simulink model "untitled2"  (R2018b)
settings: Solver=VariableStepAuto  StartTime=0.0  StopTime=3  RelTol=1e-3
libraries: commfilt2 x2, commsink2 x1, commrandsrc3 x1
settings Model: Creator=nhat  LastModifiedBy=nhat

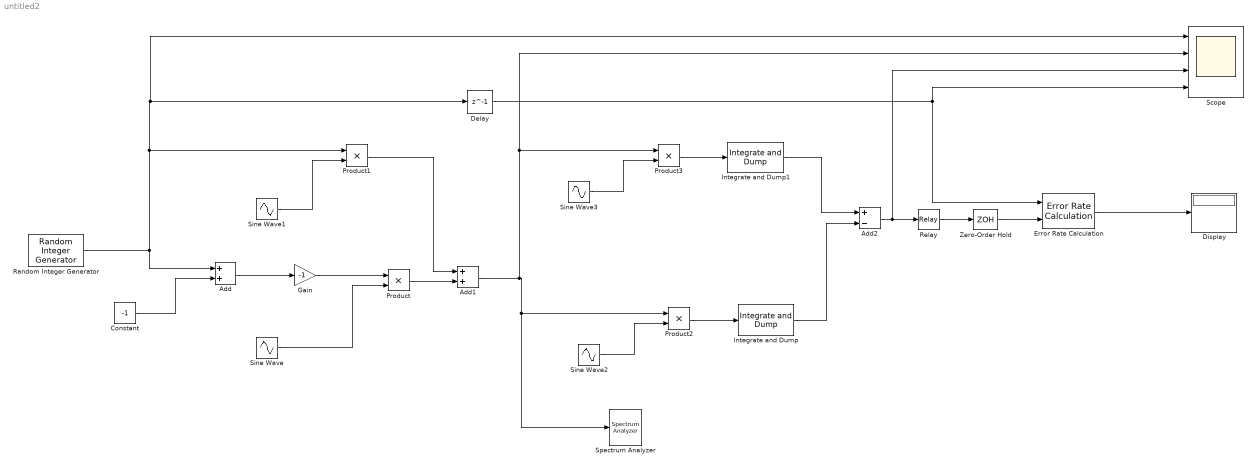
== system untitled2 ==
  Add : Sum
  Add1 : Sum
  Add2 : Sum  Inputs=+-
  Constant : Constant  Value=-1
  Delay : Delay  DelayLength=1
  Display : Display
  Error Rate Calculation : commsink2/Error Rate Calculation  N=0  st_delay=0  cp_mode=Entire frame  subframe=[]  PMode=Port  WsName=ErrorVec  RsMode2=off  stop=off  numErr=100  maxBits=1e6
  Gain : Gain  Gain=-1
  Integrate and Dump : commfilt2/Integrate and Dump  obssamples=100  offsetsamples=0  nodump=off  roundingMode=Floor  overflowMode=off  outputDataTypeStr=Inherit: Same as accumulator  outputLastDataTypeStr=Inherit: Same as accumulator
      settings: SourceProductName=Communications System Toolbox
  Integrate and Dump1 : commfilt2/Integrate and Dump  obssamples=100  offsetsamples=0  nodump=off  roundingMode=Floor  overflowMode=off  outputDataTypeStr=Inherit: Same as accumulator  outputLastDataTypeStr=Inherit: Same as accumulator
      settings: SourceProductName=Communications System Toolbox
  Product{,1..3} (4 alike) : Product
  Random Integer Generator : commrandsrc3/Random Integer Generator  SetSize=2  SeedSource=Auto  Seed=0  SampleTime=1/1000  SamplesPerFrame=1  OutputDataType=double  SimulateUsing=Interpreted execution
  Relay : Relay  OnSwitchValue=1  OffSwitchValue=0
  Scope : Scope  NumInputPorts=4
  Sine Wave : Sin  Frequency=10000*2*pi  SampleTime=1/100000
  Sine Wave1 : Sin  Frequency=15000*pi*2  SampleTime=1/100000
  Sine Wave2 : Sin  Frequency=10000*2*pi  SampleTime=1/100000
  Sine Wave3 : Sin  Frequency=15000*2*pi  SampleTime=1/100000
  Spectrum Analyzer : SpectrumAnalyzer
  Zero-Order Hold : ZeroOrderHold  SampleTime=1/1000
  wires:
  Random Integer Generator/1 -> Scope/1, Delay/1, Product1/1, Add/1
  Constant/1 -> Add/2
  Add/1 -> Gain/1
  Gain/1 -> Product/1
  Sine Wave/1 -> Product/2
  Product/1 -> Add1/2
  Sine Wave1/1 -> Product1/2
  Product1/1 -> Add1/1
  Sine Wave2/1 -> Product2/2
  Product2/1 -> Integrate and Dump/1
  Product3/1 -> Integrate and Dump1/1
  Sine Wave3/1 -> Product3/2
  Integrate and Dump1/1 -> Add2/1
  Integrate and Dump/1 -> Add2/2
  Add1/1 -> Scope/2, Product3/1, Spectrum Analyzer/1, Product2/1
  Add2/1 -> Scope/3, Relay/1
  Relay/1 -> Zero-Order Hold/1
  Zero-Order Hold/1 -> Error Rate Calculation/2
  Error Rate Calculation/1 -> Display/1
  Delay/1 -> Scope/4, Error Rate Calculation/1
